simulink model "batterydischargingcharging"  (R2014b)
settings: Solver=ode45  StartTime=0.0  StopTime=10.0  RelTol=1e-3
undefined symbols (not defined in the file): Hydride, Metal, Nickel
libraries: powerlib x8, electricdrivelib x2
settings Model: Creator=reshma  LastModifiedBy=reshma

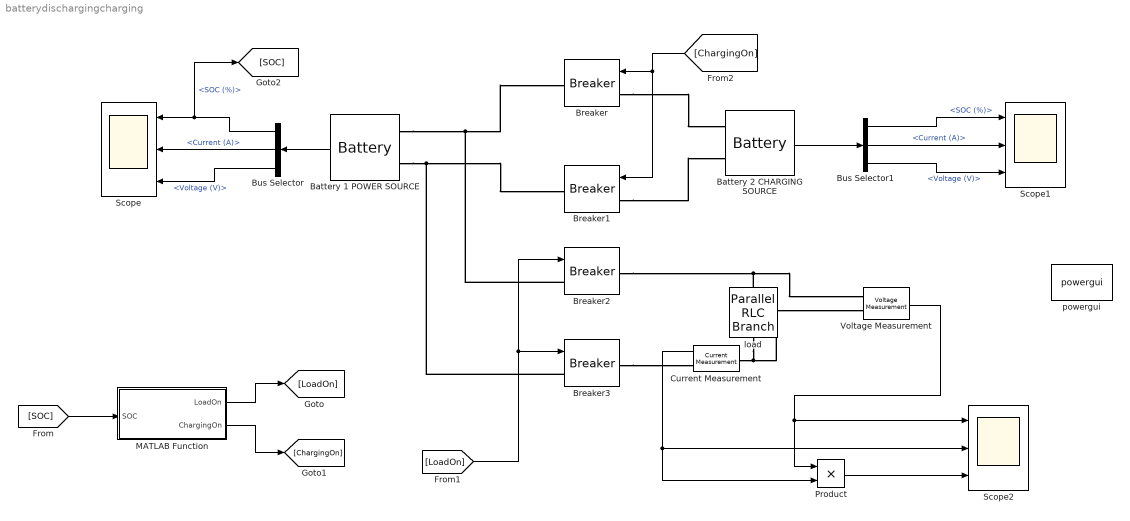
== system batterydischargingcharging ==
  Battery 1 POWER SOURCE : electricdrivelib/Extra Sources/Battery  BatType=Nickel-Metal-Hydride  ShowDetailedParameters=off  NomV=5  NomQ=1  SOC=100  PresetModel=off  MaxQ=1.0769  FullV=5.8898  Dis_rate=0.2  R=0.05  Normal_OP=0.96154  expZone="[5.4237         0.2]"  Dis_Char=off  current=[6.5 13.5 32]  Units=Ampere-hour  Batt_Tr=30
  Battery 2 CHARGING SOURCE : electricdrivelib/Extra Sources/Battery  BatType=Nickel-Metal-Hydride  ShowDetailedParameters=off  NomV=3  NomQ=0.7  SOC=50  PresetModel=on  MaxQ=0.5  FullV=2.7  Dis_rate=0.3  R=0.30769  Normal_OP=0.6  expZone="[130.1695           0.4]"  Dis_Char=off  current=[6.5 13.5 32]  Units=Ampere-hour  Batt_Tr=6000
  Breaker{,1..3} (4 alike) : powerlib/Elements/Breaker  InitialState=0  SwitchingTimes="[1/60  5/60]"  External=on  BreakerResistance=0.01  SnubberResistance=1e6  SnubberCapacitance=inf  Measurements=None  MoreParameters=on  NoBreakLoop=off
  Bus Selector : BusSelector  OutputSignals=SOC (%),Current (A),Voltage (V)
  Bus Selector1 : BusSelector  OutputSignals=SOC (%),Current (A),Voltage (V)
  Current Measurement : powerlib/Measurements/Current Measurement  PhasorSimulation=off  OutputType=Complex  PSBequivalent=0
  MATLAB Function : MATLAB Function  TreatAsAtomicUnit=on
  Product : Product
  Scope : Scope  NumInputPorts=3
      settings: YMin=-5~-5~-5  YMax=5~5~5
  Scope1 : Scope  NumInputPorts=3
      settings: YMin=-5~-5~-5  YMax=5~5~5
  Scope2 : Scope  NumInputPorts=3
      settings: YMin=-5~-5~-5  YMax=5~5~5  SaveName=ScopeData2
  Voltage Measurement : powerlib/Measurements/Voltage Measurement  PhasorSimulation=off  OutputType=Complex  PSBequivalent=0
  "load " : powerlib/Elements/Parallel RLC Branch  LConnTagsString=a  RConnTagsString=__new0  BranchType=R  Resistance=10  Inductance=1e-3  SetiL0=off  InitialCurrent=0  Capacitance=1e-6  Setx0=off  InitialVoltage=0  Measurements=None
  powergui : powerlib/powergui  Priority=1  SimulationMode=Continuous  SolverType=Tustin/Backward Euler (TBE)  SampleTime=50e-6  frequency=60  SPID=off  DisableSnubberDevices=off  DisableRonSwitches=off  DisableVfSwitches=off  SwTol=0  DisplayEquations=off  Interpol=off  methode=off  Ts=100  frequencyindice=0  Pbase=100e6  ErrMax=1e-4  Iterations=50  UnitsV=kV  UnitsW=MW  FunctionMessages=off  echomessages=off  HookPort=off  EnableUseOfTLC=off  x0status=blocks  RestoreLinks=warning  ResistiveCurrentMeasurement=off  Frange=[0:2:500]  Ylog=off  Xlog=on  ShowGrid=off  save=off  variable=ZData  structure=0  ZoomFFT=off  StartTime=0.0  cycles=1  DisplayStyle=1  fundamental=60  FreqAxis=off  MaxFrequency=1000  frequencyindicesteady=1  RmsSteady=1  display=off
  wires:
  Battery 1 POWER SOURCE/1 -> Bus Selector/1
  Bus Selector/2 -> Scope/2  "<Current (A)>"
  Bus Selector/3 -> Scope/3  "<Voltage (V)>"
  Bus Selector/1 -> [SOC], Scope/1  "<SOC (%)>"
  Battery 2 CHARGING SOURCE/1 -> Bus Selector1/1
  Bus Selector1/1 -> Scope1/1  "<SOC (%)>"
  Bus Selector1/2 -> Scope1/2  "<Current (A)>"
  Bus Selector1/3 -> Scope1/3  "<Voltage (V)>"
  [SOC] -> MATLAB Function/1(SOC)
  MATLAB Function/1(LoadOn) -> [LoadOn]
  MATLAB Function/2(ChargingOn) -> [ChargingOn]
  [ChargingOn] -> Breaker/1, Breaker1/1
  [LoadOn] -> Breaker2/1, Breaker3/1
  Product/1 -> Scope2/3
  Current Measurement/1 -> Scope2/2, Product/2
  Voltage Measurement/1 -> Product/1, Scope2/1
  connections:
  Battery 1 POWER SOURCE/LConn1 -- Breaker2/LConn1 -- Breaker/RConn1
  Battery 1 POWER SOURCE/LConn2 -- Breaker3/LConn1 -- Breaker1/RConn1
  Breaker/LConn1 -- Battery 2 CHARGING SOURCE/LConn1
  Breaker1/LConn1 -- Battery 2 CHARGING SOURCE/LConn2
  Breaker2/RConn1 -- "load "/RConn1 -- Voltage Measurement/LConn1
  Current Measurement/LConn1 -- Voltage Measurement/LConn2 -- "load "/LConn1
  Breaker3/RConn1 -- Current Measurement/RConn1

== matlab function batterydischargingcharging/MATLAB Function ==
  data: SOC input; LoadOn output; ChargingOn output
function [LoadOn, ChargingOn] = fcn(SOC)
%#codegen
LoadOn=1;
ChargingOn=0;
if (SOC>=80)
    LoadOn=1;
ChargingOn=0;
end

if (SOC<40)
    LoadOn=0;
ChargingOn=1;

end
